simulink model "grapebot_sim_bridge"  (R2024b)
settings: Solver=FixedStepDiscrete  StartTime=0.0  StopTime=Inf  FixedStep=0.02  RelTol=1e-3
InitFcn:
  | clc,clear
  | 
  | rosgenmsg(".")
  | 
  | addpath(genpath("./matlab_msg_gen_ros1"))
  | 
  | % clear classes
  | % rehash toolboxcache
StopFcn:
  | if ros.internal.Global.isNodeActive
  |     rosshutdown;
  | end
undefined symbols (not defined in the file or in its folder): Angular, Linear
libraries: robotlib x3
settings Model: Creator=peng  LastModifiedBy=peng
settings OptimizationCC: DefaultParameterBehavior=Inlined  EnhancedBackFolding=on  PassReuseOutputArgsAs=Individual arguments  ZeroExternalMemoryAtStartup=off  ZeroInternalMemoryAtStartup=off  MaxStackSize=64  OptimizeBlockOrder=speed  DifferentSizesBufferReuse=on  OptimizationCustomize=off  EfficientTunableParamExpr=on
settings DebuggingCC: ParameterTunabilityLossMsg=error
settings HardwareCC: ProdBitPerPointer=32  ProdBitPerSizeT=32  ProdBitPerPtrDiffT=32  ProdLargestAtomicFloat=None  ProdIntDivRoundTo=Undefined  ProdEndianess=Unspecified  ProdWordSize=32  ProdHWDeviceType=Generic->Unspecified (assume 32-bit Generic)  UseEmbeddedCoderFeatures=off
settings RTWCC: Description=Embedded Coder  SystemTargetFile=ert.tlc  HardwareBoard=Robot Operating System (ROS)  TLCOptions="-aInlineSetEventsForThisBaseRateFcn=TLC_FALSE -aSuppressMultiTaskScheduler=TLC_FALSE  -aRateBasedStepFcn=0"  TemplateMakefile=ert_default_tmf  Toolchain=Catkin  TargetLang=C++
settings CodeAppCC: ForceParamTrailComments=on  IgnoreCustomStorageClasses=off  OperatorAnnotations=on  SimulinkDataObjDesc=on  SFDataObjDesc=on  InsertBlockDesc=on
settings ERTTargetCC: SupportNonInlinedSFcns=on

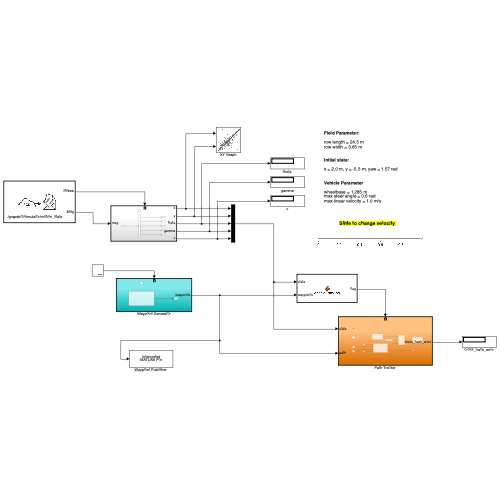
[thumbnail: Simulink's stored preview of the top-level diagram]
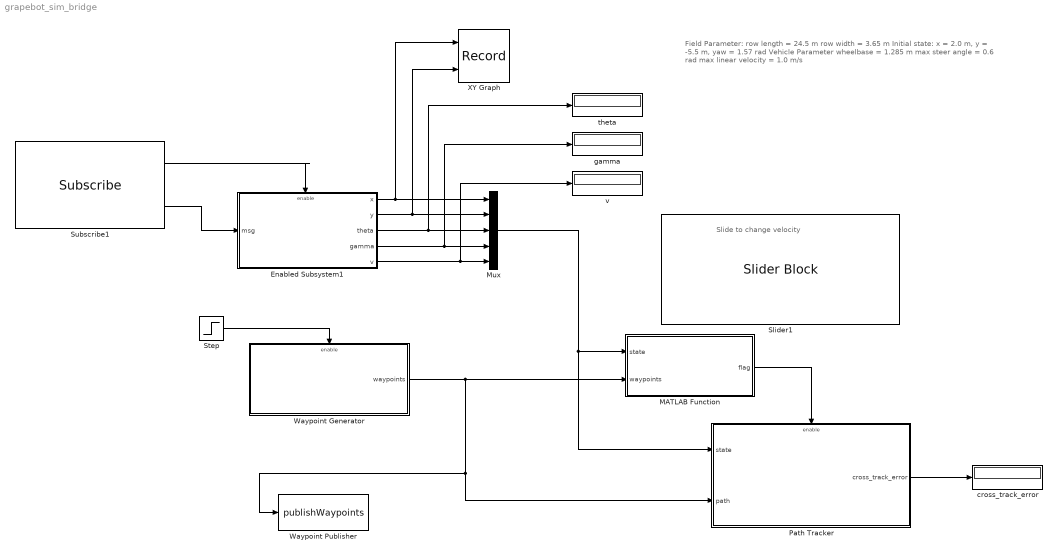
== system grapebot_sim_bridge ==
  note: Slide to change velocity
  note: Field Parameter:
      |
      | row length = 24.5 m
      | row width = 3.65 m
      |
      | Initial state:
      |
      | x = 2.0 m, y = -5.5 m, yaw = 1.57 rad
      |
      | Vehicle Parameter
      |
      | wheelbase = 1.285 m
      | max steer angle = 0.6 rad
      | max linear velocity = 1.0 m/s
  Enabled Subsystem1 : Subsystem  TreatAsAtomicUnit=on
  MATLAB Function : MATLAB Function  TreatAsAtomicUnit=on
  Mux : Mux  Inputs=5
  Path Tracker : Subsystem  TreatAsAtomicUnit=on
  Slider1 : SliderBlock  LabelPosition=Hide  ScaleMin=0.0  ScaleMax=1.0  TickInterval=0.2
  Step : Step  Time=0.01  Before=1  After=0
  Subscribe1 : robotlib/Subscribe  topicSource=Select from ROS network  topic=/grapebot/simulator/motion_state  messageType=robot_msgs/MotionState  SampleTime=0.02  legacyBusStruct=off  messageQueueLength=1
  Waypoint Generator : Subsystem  TreatAsAtomicUnit=on
  "Waypoint Publisher " : MATLABFcn  StartFcn=rosinit  StopFcn=rosshutdown  MATLABFcn=publishWaypoints  OutputDimensions=0
  XY Graph : Record  FileSettingsInternal="{\"entries\":[{\"content\":{\"excelSettings\":{\"content\":{},\"type\":\"Streamout.ExcelSettings\"}},\"type\":\"Streamout.FileSettingStorage\",\"uuid\":\"\"}],\"packageUris\":[\"http:\\/\\/schema.mathworks.com\\/mf0\\/streamout_blocks\\/R2020a\"],\"version\":\"1.0\"}"  Layout=[1 1]  SignalsInternal="{\"entries\":[{\"content\":{\"signals\":[{\"content\":{\"blockPath\":[],\"dimensions\":[1],\"domain\":\"\",\"lineColor\":\"#ff6929\",\"lineWidth\":2,\"port\":1,\"sid\":[\"\"],\"signalID\":1,\"signalName\":\"Enabled\\nSubsystem1:1\"},\"type\":\"RecordBlkView.Signal\",\"uuid\":\"\"},{\"content\":{\"blockPath\":[],\"dimensions\":[1],\"domain\":\"\",\"lineColor\":\"#b746ff\",\"lineWidth\":2,\"port\":2,\"sid\":[\"\"],\"signalID\":2,\"signalName\":\"Enabled\\nSubsystem1:2\"},\"type\":\"RecordBlkView.Signal\",\"uuid\":\"\"}]},\"type\":\"RecordBlkView.InputSignals\",\"uuid\":\"\"}],\"packageUris\":[\"http:\\/\\/schema.mathworks.com\\/mf0\\/streamout_blocks\\/R2020a\"],\"version\":\"1.0\"}"  VisualizationBindings="{\"xyplotplugin\":{\"info\":[{\"series\":[],\"subplotID\":1}]}}"  CompatibilityTag=XY
  cross_track_error : Display
  gamma : Display
  theta : Display
  v : Display
  wires:
  Enabled Subsystem1/1(x) -> Mux/1, XY Graph/1
  Enabled Subsystem1/2(y) -> Mux/2, XY Graph/2
  Enabled Subsystem1/3(theta) -> theta/1, Mux/3
  Enabled Subsystem1/4(gamma) -> Mux/4, gamma/1
  Enabled Subsystem1/5(v) -> Mux/5, v/1
  MATLAB Function/1(flag) -> Path Tracker/Enable
  Waypoint Generator/1(waypoints) -> "Waypoint Publisher "/1, Path Tracker/2(path), MATLAB Function/2(waypoints)
  Step/1 -> Waypoint Generator/Enable
  Path Tracker/1(cross_track_error) -> cross_track_error/1
  Subscribe1/1 -> Enabled Subsystem1/Enable
  Subscribe1/2 -> Enabled Subsystem1/1(msg)
  Mux/1 -> MATLAB Function/1(state), Path Tracker/1(state)

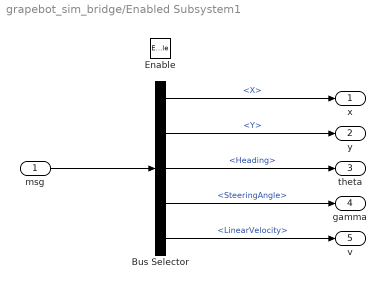
== system grapebot_sim_bridge/Enabled Subsystem1 ==
  msg : Inport
  Enable : EnablePort
  Bus Selector : BusSelector  OutputSignals=X,Y,Heading,SteeringAngle,LinearVelocity
  x : Outport
  y : Outport  Port=2
  theta : Outport  Port=3
  gamma : Outport  Port=4
  v : Outport  Port=5
  wires:
  msg/1 -> Bus Selector/1
  Bus Selector/1 -> x/1  "<X>"
  Bus Selector/2 -> y/1  "<Y>"
  Bus Selector/3 -> theta/1  "<Heading>"
  Bus Selector/4 -> gamma/1  "<SteeringAngle>"
  Bus Selector/5 -> v/1  "<LinearVelocity>"

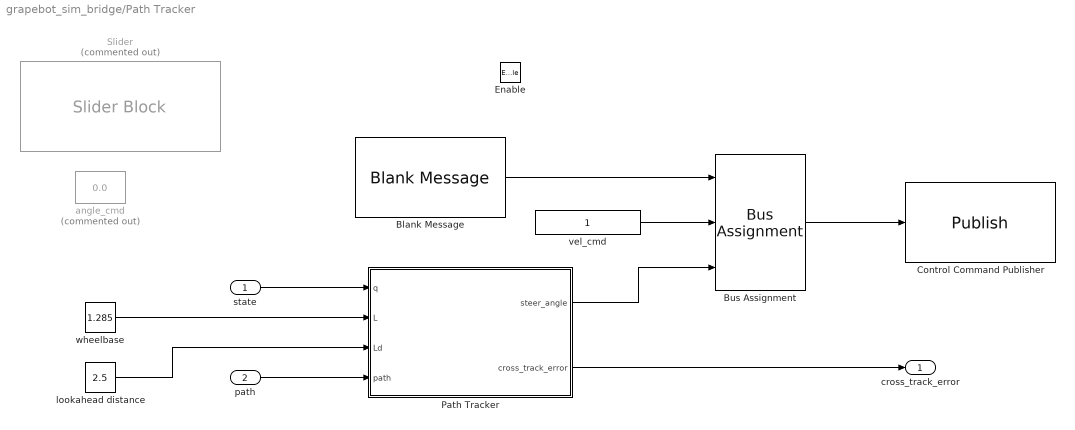
== system grapebot_sim_bridge/Path Tracker ==
  state : Inport
  path : Inport  Port=2
  Enable : EnablePort
  Blank Message : robotlib/Blank Message  messageClass=Message  entityType=geometry_msgs/Twist  messageType=geometry_msgs/Twist  SampleTime=-1  legacyBusStruct=off
  Bus Assignment : BusAssignment  AssignedSignals=Linear.X,Angular.Z
  Control Command Publisher : robotlib/Publish  topicSource=Select from ROS network  topic=/grapebot/matlab/cmd_vel  messageType=geometry_msgs/Twist  legacyBusStruct=off  messageQueueLength=1
  Path Tracker : MATLAB Function  TreatAsAtomicUnit=on
  Slider : SliderBlock  Commented=on  ScaleMin=-0.5  ScaleMax=0.5
  angle_cmd : Constant  Commented=on  Value=0.0
  lookahead distance : Constant  Value=2.5
  vel_cmd : Constant
  wheelbase : Constant  Value=1.285  SampleTime=Inf
  cross_track_error : Outport
  wires:
  Path Tracker/1(steer_angle) -> Bus Assignment/3
  Path Tracker/2(cross_track_error) -> cross_track_error/1
  vel_cmd/1 -> Bus Assignment/2
  Bus Assignment/1 -> Control Command Publisher/1
  Blank Message/1 -> Bus Assignment/1
  wheelbase/1 -> Path Tracker/2(L)
  lookahead distance/1 -> Path Tracker/3(Ld)
  path/1 -> Path Tracker/4(path)
  state/1 -> Path Tracker/1(q)

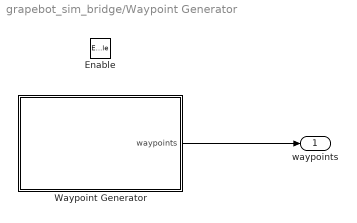
== system grapebot_sim_bridge/Waypoint Generator ==
  Enable : EnablePort
  Waypoint Generator : MATLAB Function  TreatAsAtomicUnit=on  SystemSampleTime=1
  waypoints : Outport
  wires:
  Waypoint Generator/1(waypoints) -> waypoints/1

== matlab function grapebot_sim_bridge/Waypoint Generator/Waypoint Generator ==
  data: waypoints output
function waypoints = waypointGenerator()

% ---------------------------------------------------------------
% NOTE: The following code is provided only for testing purposes. 
%       Comment it out after adding your own implementation.
data = load("test_wpts.mat", "wpts");
waypoints = data.wpts;
%
% ---------------------------------------------------------------

%%%%%%%%%%%%%%%%%%
% Insert your code here



%%%%%%%%%%%%%%%%%%

plant_bed = load("plant_bed.mat", "PLANT_BED_D", "PLANT_BED_F");
start_state = [2.0, -5.5, 1.57];

hold on
scatter(start_state(1), start_state(2), 30, "*b")

for i=1:length(plant_bed.PLANT_BED_D)
    plot([plant_bed.PLANT_BED_D(1, i), plant_bed.PLANT_BED_F(1, i)],...
         [plant_bed.PLANT_BED_D(2, i), plant_bed.PLANT_BED_F(2, i)],...
         'r', 'LineWidth', 1.5)
end

plot(waypoints(1,:), waypoints(2,:), '-og')
hold off

end

== matlab function grapebot_sim_bridge/Path Tracker/Path Tracker ==
  data: q input; steer_angle output; L input; Ld input; path input; cross_track_error output
function [steer_angle, cross_track_error] = purePursuitController(q, L, Ld, path)
% Pure Pursuit controller %
% state is 
    % q(1) -> x
    % q(2) -> y
    % q(3) -> theta (orientation in world frame)
    % q(4) -> gamma (steering angle)
    % q(5) -> v (linear velocity)

% L is the wheelbase
% Ld is the look-ahead distance
% path is a 2xN array of N waypoints in the world frame


% ---------------------------------------------------------------
% NOTE: The following code is provided only for testing purposes. 
%       Comment it out after adding your own implementation.
x     = q(1);
y     = q(2);
theta = q(3);

N = size(path,2);

dx = path(1,:) - x;
dy = path(2,:) - y;
d2 = dx.^2 + dy.^2;
[~, idx_closest] = min(d2);

idx_target = idx_closest;

while idx_target < N && sqrt((path(1,idx_target)-x)^2 + (path(2,idx_target)-y)^2) < Ld
    idx_target = idx_target + 1;
end

idx_target = min(idx_target, N);

xt = path(1,idx_target);
yt = path(2,idx_target);

dx_t =  xt - x;
dy_t =  yt - y;

alpha = wrapToPi(atan2(dy_t,dx_t) - theta);

steer_angle = atan2(2*L*sin(alpha), Ld);

if idx_closest < N
    p1 = path(:,idx_closest);
    p2 = path(:,idx_closest+1);

    v_seg = p2 - p1;
    v_pt  = [x; y] - p1;
    t = dot(v_pt,v_seg)/dot(v_seg,v_seg);
    proj = p1 + t*v_seg;

    e_vec = [x; y] - proj;
    cross_track_error = sign( v_seg(1)*e_vec(2) - v_seg(2)*e_vec(1) ) * norm(e_vec);
else

    cross_track_error = sign( dx(end)*dy(end) ) * sqrt(d2(idx_closest));
end
% ---------------------------------------------------------------


%%%%%%%%%%%%%%%%%%%%
% Insert your code here


%%%%%%%%%%%%%%%%%%%%

end

== matlab function grapebot_sim_bridge/MATLAB Function ==
  data: state input; waypoints input; flag output
function flag = enableTracking(state, waypoints)

threshold = 1.5;

current_xy = [state(1); state(2)];
distance = norm(current_xy - waypoints(:, end));

persistent has_reached
if isempty(has_reached)
    has_reached = false;
end

if distance < threshold
    has_reached = true;
end

if has_reached
    flag = -1;
else
    flag = 1;
end
